simulink model "BaseEngineController_LS"  (Simulink 7.7)
settings: Solver=FixedStepDiscrete  StartTime=0.0  StopTime=10.0  RelTol=1e-3
PreLoadFcn:
  | try, eval([bdroot '_setup']); catch, eval('model_setup', ''); end
InitFcn:
  | try, eval([bdroot '_setup']); catch, eval('model_setup', ''); end
undefined symbols (not defined in the file): ECU555, High, motohawk_build_version, motohawk_trunc_name, motohawk_vardec_config_group, motohawk_vardec_path, True
libraries: MotoHawk_lib x1418, motohawk_control_primitives_lib x183, motohawk_engine_lib x32, simulink x21, motohawk_annotations_lib x9, AutoDoc_lib x8, simulink_extras x4, motohawk_ccp_examples_lib x1, motohawk_control_primitives_motoshare_lib x1
(part 19 of 27)

== system BaseEngineController_LS/Foreground/Control/ActuatorCharacterization/SequenceCutPattern/Hard Cycle Cut Pattern/Cycle4CutPatter ==
  Mux1 : Mux  Inputs=8
  motohawk_calibration10 : MotoHawk_lib/Calibration & Probing Blocks/motohawk_calibration  nam='HardCycle4Cyl4'  val=0  storage=Calibration  show_more=on  name_source=Use Parameter  data_type=int8  read_level=1  write_level=1  ovr_cals=on  view_as=Enumeration  enum_struct={'Enable', 'Cut'}  vector_style=Wide Row  use_help_units=on  help=''  units=''  use_header_enum=off  row_header_enum={}  col_header_enum={}  use_min_max=off  min_val=-inf  max_val=inf  use_precision=off  precision=''  gain=1  offset=0  exp=1  use_mototune_group=on  mototune_group=motohawk_vardec_path(gcb)
  motohawk_calibration11 : MotoHawk_lib/Calibration & Probing Blocks/motohawk_calibration  nam='HardCycle4Cyl1'  val=1  storage=Calibration  show_more=on  name_source=Use Parameter  data_type=int8  read_level=1  write_level=1  ovr_cals=on  view_as=Enumeration  enum_struct={'Enable', 'Cut'}  vector_style=Wide Row  use_help_units=on  help=''  units=''  use_header_enum=off  row_header_enum={}  col_header_enum={}  use_min_max=off  min_val=-inf  max_val=inf  use_precision=off  precision=''  gain=1  offset=0  exp=1  use_mototune_group=on  mototune_group=motohawk_vardec_path(gcb)
  motohawk_calibration12 : MotoHawk_lib/Calibration & Probing Blocks/motohawk_calibration  nam='HardCycle4Cyl5'  val=1  storage=Calibration  show_more=on  name_source=Use Parameter  data_type=int8  read_level=1  write_level=1  ovr_cals=on  view_as=Enumeration  enum_struct={'Enable', 'Cut'}  vector_style=Wide Row  use_help_units=on  help=''  units=''  use_header_enum=off  row_header_enum={}  col_header_enum={}  use_min_max=off  min_val=-inf  max_val=inf  use_precision=off  precision=''  gain=1  offset=0  exp=1  use_mototune_group=on  mototune_group=motohawk_vardec_path(gcb)
  motohawk_calibration13 : MotoHawk_lib/Calibration & Probing Blocks/motohawk_calibration  nam='HardCycle4Cyl6'  val=1  storage=Calibration  show_more=on  name_source=Use Parameter  data_type=int8  read_level=1  write_level=1  ovr_cals=on  view_as=Enumeration  enum_struct={'Enable', 'Cut'}  vector_style=Wide Row  use_help_units=on  help=''  units=''  use_header_enum=off  row_header_enum={}  col_header_enum={}  use_min_max=off  min_val=-inf  max_val=inf  use_precision=off  precision=''  gain=1  offset=0  exp=1  use_mototune_group=on  mototune_group=motohawk_vardec_path(gcb)
  motohawk_calibration14 : MotoHawk_lib/Calibration & Probing Blocks/motohawk_calibration  nam='HardCycle4Cyl7'  val=1  storage=Calibration  show_more=on  name_source=Use Parameter  data_type=int8  read_level=1  write_level=1  ovr_cals=on  view_as=Enumeration  enum_struct={'Enable', 'Cut'}  vector_style=Wide Row  use_help_units=on  help=''  units=''  use_header_enum=off  row_header_enum={}  col_header_enum={}  use_min_max=off  min_val=-inf  max_val=inf  use_precision=off  precision=''  gain=1  offset=0  exp=1  use_mototune_group=on  mototune_group=motohawk_vardec_path(gcb)
  motohawk_calibration15 : MotoHawk_lib/Calibration & Probing Blocks/motohawk_calibration  nam='HardCycle4Cyl8'  val=1  storage=Calibration  show_more=on  name_source=Use Parameter  data_type=int8  read_level=1  write_level=1  ovr_cals=on  view_as=Enumeration  enum_struct={'Enable', 'Cut'}  vector_style=Wide Row  use_help_units=on  help=''  units=''  use_header_enum=off  row_header_enum={}  col_header_enum={}  use_min_max=off  min_val=-inf  max_val=inf  use_precision=off  precision=''  gain=1  offset=0  exp=1  use_mototune_group=on  mototune_group=motohawk_vardec_path(gcb)
  motohawk_calibration8 : MotoHawk_lib/Calibration & Probing Blocks/motohawk_calibration  nam='HardCycle4Cyl2'  val=1  storage=Calibration  show_more=on  name_source=Use Parameter  data_type=int8  read_level=1  write_level=1  ovr_cals=on  view_as=Enumeration  enum_struct={'Enable', 'Cut'}  vector_style=Wide Row  use_help_units=on  help=''  units=''  use_header_enum=off  row_header_enum={}  col_header_enum={}  use_min_max=off  min_val=-inf  max_val=inf  use_precision=off  precision=''  gain=1  offset=0  exp=1  use_mototune_group=on  mototune_group=motohawk_vardec_path(gcb)
  motohawk_calibration9 : MotoHawk_lib/Calibration & Probing Blocks/motohawk_calibration  nam='HardCycle4Cyl3'  val=1  storage=Calibration  show_more=on  name_source=Use Parameter  data_type=int8  read_level=1  write_level=1  ovr_cals=on  view_as=Enumeration  enum_struct={'Enable', 'Cut'}  vector_style=Wide Row  use_help_units=on  help=''  units=''  use_header_enum=off  row_header_enum={}  col_header_enum={}  use_min_max=off  min_val=-inf  max_val=inf  use_precision=off  precision=''  gain=1  offset=0  exp=1  use_mototune_group=on  mototune_group=motohawk_vardec_path(gcb)
  Out : Outport
  wires:
  Mux1/1 -> Out/1
  motohawk_calibration15/1 -> Mux1/8
  motohawk_calibration14/1 -> Mux1/7
  motohawk_calibration13/1 -> Mux1/6
  motohawk_calibration12/1 -> Mux1/5
  motohawk_calibration10/1 -> Mux1/4
  motohawk_calibration9/1 -> Mux1/3
  motohawk_calibration8/1 -> Mux1/2
  motohawk_calibration11/1 -> Mux1/1

== system BaseEngineController_LS/Foreground/Control/ActuatorCharacterization/SequenceCutPattern/Medium Cycle Cut Pattern/Cycle1CutPatter ==
  Mux1 : Mux  Inputs=8
  motohawk_calibration10 : MotoHawk_lib/Calibration & Probing Blocks/motohawk_calibration  nam='MediumCycle1Cyl4'  val=0  storage=Calibration  show_more=on  name_source=Use Parameter  data_type=int8  read_level=1  write_level=1  ovr_cals=on  view_as=Enumeration  enum_struct={'Enable', 'Cut'}  vector_style=Wide Row  use_help_units=on  help=''  units=''  use_header_enum=off  row_header_enum={}  col_header_enum={}  use_min_max=off  min_val=-inf  max_val=inf  use_precision=off  precision=''  gain=1  offset=0  exp=1  use_mototune_group=on  mototune_group=motohawk_vardec_path(gcb)
  motohawk_calibration11 : MotoHawk_lib/Calibration & Probing Blocks/motohawk_calibration  nam='MediumCycle1Cyl1'  val=1  storage=Calibration  show_more=on  name_source=Use Parameter  data_type=int8  read_level=1  write_level=1  ovr_cals=on  view_as=Enumeration  enum_struct={'Enable', 'Cut'}  vector_style=Wide Row  use_help_units=on  help=''  units=''  use_header_enum=off  row_header_enum={}  col_header_enum={}  use_min_max=off  min_val=-inf  max_val=inf  use_precision=off  precision=''  gain=1  offset=0  exp=1  use_mototune_group=on  mototune_group=motohawk_vardec_path(gcb)
  motohawk_calibration12 : MotoHawk_lib/Calibration & Probing Blocks/motohawk_calibration  nam='MediumCycle1Cyl5'  val=1  storage=Calibration  show_more=on  name_source=Use Parameter  data_type=int8  read_level=1  write_level=1  ovr_cals=on  view_as=Enumeration  enum_struct={'Enable', 'Cut'}  vector_style=Wide Row  use_help_units=on  help=''  units=''  use_header_enum=off  row_header_enum={}  col_header_enum={}  use_min_max=off  min_val=-inf  max_val=inf  use_precision=off  precision=''  gain=1  offset=0  exp=1  use_mototune_group=on  mototune_group=motohawk_vardec_path(gcb)
  motohawk_calibration13 : MotoHawk_lib/Calibration & Probing Blocks/motohawk_calibration  nam='MediumCycle1Cyl6'  val=1  storage=Calibration  show_more=on  name_source=Use Parameter  data_type=int8  read_level=1  write_level=1  ovr_cals=on  view_as=Enumeration  enum_struct={'Enable', 'Cut'}  vector_style=Wide Row  use_help_units=on  help=''  units=''  use_header_enum=off  row_header_enum={}  col_header_enum={}  use_min_max=off  min_val=-inf  max_val=inf  use_precision=off  precision=''  gain=1  offset=0  exp=1  use_mototune_group=on  mototune_group=motohawk_vardec_path(gcb)
  motohawk_calibration14 : MotoHawk_lib/Calibration & Probing Blocks/motohawk_calibration  nam='MediumCycle1Cyl7'  val=1  storage=Calibration  show_more=on  name_source=Use Parameter  data_type=int8  read_level=1  write_level=1  ovr_cals=on  view_as=Enumeration  enum_struct={'Enable', 'Cut'}  vector_style=Wide Row  use_help_units=on  help=''  units=''  use_header_enum=off  row_header_enum={}  col_header_enum={}  use_min_max=off  min_val=-inf  max_val=inf  use_precision=off  precision=''  gain=1  offset=0  exp=1  use_mototune_group=on  mototune_group=motohawk_vardec_path(gcb)
  motohawk_calibration15 : MotoHawk_lib/Calibration & Probing Blocks/motohawk_calibration  nam='MediumCycle1Cyl8'  val=1  storage=Calibration  show_more=on  name_source=Use Parameter  data_type=int8  read_level=1  write_level=1  ovr_cals=on  view_as=Enumeration  enum_struct={'Enable', 'Cut'}  vector_style=Wide Row  use_help_units=on  help=''  units=''  use_header_enum=off  row_header_enum={}  col_header_enum={}  use_min_max=off  min_val=-inf  max_val=inf  use_precision=off  precision=''  gain=1  offset=0  exp=1  use_mototune_group=on  mototune_group=motohawk_vardec_path(gcb)
  motohawk_calibration8 : MotoHawk_lib/Calibration & Probing Blocks/motohawk_calibration  nam='MediumCycle1Cyl2'  val=1  storage=Calibration  show_more=on  name_source=Use Parameter  data_type=int8  read_level=1  write_level=1  ovr_cals=on  view_as=Enumeration  enum_struct={'Enable', 'Cut'}  vector_style=Wide Row  use_help_units=on  help=''  units=''  use_header_enum=off  row_header_enum={}  col_header_enum={}  use_min_max=off  min_val=-inf  max_val=inf  use_precision=off  precision=''  gain=1  offset=0  exp=1  use_mototune_group=on  mototune_group=motohawk_vardec_path(gcb)
  motohawk_calibration9 : MotoHawk_lib/Calibration & Probing Blocks/motohawk_calibration  nam='MediumCycle1Cyl3'  val=0  storage=Calibration  show_more=on  name_source=Use Parameter  data_type=int8  read_level=1  write_level=1  ovr_cals=on  view_as=Enumeration  enum_struct={'Enable', 'Cut'}  vector_style=Wide Row  use_help_units=on  help=''  units=''  use_header_enum=off  row_header_enum={}  col_header_enum={}  use_min_max=off  min_val=-inf  max_val=inf  use_precision=off  precision=''  gain=1  offset=0  exp=1  use_mototune_group=on  mototune_group=motohawk_vardec_path(gcb)
  Out : Outport
  wires:
  Mux1/1 -> Out/1
  motohawk_calibration15/1 -> Mux1/8
  motohawk_calibration14/1 -> Mux1/7
  motohawk_calibration13/1 -> Mux1/6
  motohawk_calibration12/1 -> Mux1/5
  motohawk_calibration10/1 -> Mux1/4
  motohawk_calibration9/1 -> Mux1/3
  motohawk_calibration8/1 -> Mux1/2
  motohawk_calibration11/1 -> Mux1/1

== system BaseEngineController_LS/Foreground/Control/ActuatorCharacterization/SequenceCutPattern/Medium Cycle Cut Pattern/Cycle2CutPatter ==
  Mux1 : Mux  Inputs=8
  motohawk_calibration10 : MotoHawk_lib/Calibration & Probing Blocks/motohawk_calibration  nam='MediumCycle2Cyl4'  val=1  storage=Calibration  show_more=on  name_source=Use Parameter  data_type=int8  read_level=1  write_level=1  ovr_cals=on  view_as=Enumeration  enum_struct={'Enable', 'Cut'}  vector_style=Wide Row  use_help_units=on  help=''  units=''  use_header_enum=off  row_header_enum={}  col_header_enum={}  use_min_max=off  min_val=-inf  max_val=inf  use_precision=off  precision=''  gain=1  offset=0  exp=1  use_mototune_group=on  mototune_group=motohawk_vardec_path(gcb)
  motohawk_calibration11 : MotoHawk_lib/Calibration & Probing Blocks/motohawk_calibration  nam='MediumCycle2Cyl1'  val=0  storage=Calibration  show_more=on  name_source=Use Parameter  data_type=int8  read_level=1  write_level=1  ovr_cals=on  view_as=Enumeration  enum_struct={'Enable', 'Cut'}  vector_style=Wide Row  use_help_units=on  help=''  units=''  use_header_enum=off  row_header_enum={}  col_header_enum={}  use_min_max=off  min_val=-inf  max_val=inf  use_precision=off  precision=''  gain=1  offset=0  exp=1  use_mototune_group=on  mototune_group=motohawk_vardec_path(gcb)
  motohawk_calibration12 : MotoHawk_lib/Calibration & Probing Blocks/motohawk_calibration  nam='MediumCycle2Cyl5'  val=1  storage=Calibration  show_more=on  name_source=Use Parameter  data_type=int8  read_level=1  write_level=1  ovr_cals=on  view_as=Enumeration  enum_struct={'Enable', 'Cut'}  vector_style=Wide Row  use_help_units=on  help=''  units=''  use_header_enum=off  row_header_enum={}  col_header_enum={}  use_min_max=off  min_val=-inf  max_val=inf  use_precision=off  precision=''  gain=1  offset=0  exp=1  use_mototune_group=on  mototune_group=motohawk_vardec_path(gcb)
  motohawk_calibration13 : MotoHawk_lib/Calibration & Probing Blocks/motohawk_calibration  nam='MediumCycle2Cyl6'  val=1  storage=Calibration  show_more=on  name_source=Use Parameter  data_type=int8  read_level=1  write_level=1  ovr_cals=on  view_as=Enumeration  enum_struct={'Enable', 'Cut'}  vector_style=Wide Row  use_help_units=on  help=''  units=''  use_header_enum=off  row_header_enum={}  col_header_enum={}  use_min_max=off  min_val=-inf  max_val=inf  use_precision=off  precision=''  gain=1  offset=0  exp=1  use_mototune_group=on  mototune_group=motohawk_vardec_path(gcb)
  motohawk_calibration14 : MotoHawk_lib/Calibration & Probing Blocks/motohawk_calibration  nam='MediumCycle2Cyl7'  val=1  storage=Calibration  show_more=on  name_source=Use Parameter  data_type=int8  read_level=1  write_level=1  ovr_cals=on  view_as=Enumeration  enum_struct={'Enable', 'Cut'}  vector_style=Wide Row  use_help_units=on  help=''  units=''  use_header_enum=off  row_header_enum={}  col_header_enum={}  use_min_max=off  min_val=-inf  max_val=inf  use_precision=off  precision=''  gain=1  offset=0  exp=1  use_mototune_group=on  mototune_group=motohawk_vardec_path(gcb)
  motohawk_calibration15 : MotoHawk_lib/Calibration & Probing Blocks/motohawk_calibration  nam='MediumCycle2Cyl8'  val=1  storage=Calibration  show_more=on  name_source=Use Parameter  data_type=int8  read_level=1  write_level=1  ovr_cals=on  view_as=Enumeration  enum_struct={'Enable', 'Cut'}  vector_style=Wide Row  use_help_units=on  help=''  units=''  use_header_enum=off  row_header_enum={}  col_header_enum={}  use_min_max=off  min_val=-inf  max_val=inf  use_precision=off  precision=''  gain=1  offset=0  exp=1  use_mototune_group=on  mototune_group=motohawk_vardec_path(gcb)
  motohawk_calibration8 : MotoHawk_lib/Calibration & Probing Blocks/motohawk_calibration  nam='MediumCycle2Cyl2'  val=0  storage=Calibration  show_more=on  name_source=Use Parameter  data_type=int8  read_level=1  write_level=1  ovr_cals=on  view_as=Enumeration  enum_struct={'Enable', 'Cut'}  vector_style=Wide Row  use_help_units=on  help=''  units=''  use_header_enum=off  row_header_enum={}  col_header_enum={}  use_min_max=off  min_val=-inf  max_val=inf  use_precision=off  precision=''  gain=1  offset=0  exp=1  use_mototune_group=on  mototune_group=motohawk_vardec_path(gcb)
  motohawk_calibration9 : MotoHawk_lib/Calibration & Probing Blocks/motohawk_calibration  nam='MediumCycle2Cyl3'  val=1  storage=Calibration  show_more=on  name_source=Use Parameter  data_type=int8  read_level=1  write_level=1  ovr_cals=on  view_as=Enumeration  enum_struct={'Enable', 'Cut'}  vector_style=Wide Row  use_help_units=on  help=''  units=''  use_header_enum=off  row_header_enum={}  col_header_enum={}  use_min_max=off  min_val=-inf  max_val=inf  use_precision=off  precision=''  gain=1  offset=0  exp=1  use_mototune_group=on  mototune_group=motohawk_vardec_path(gcb)
  Out : Outport
  wires:
  motohawk_calibration11/1 -> Mux1/1
  motohawk_calibration8/1 -> Mux1/2
  motohawk_calibration9/1 -> Mux1/3
  motohawk_calibration10/1 -> Mux1/4
  motohawk_calibration12/1 -> Mux1/5
  motohawk_calibration13/1 -> Mux1/6
  motohawk_calibration14/1 -> Mux1/7
  motohawk_calibration15/1 -> Mux1/8
  Mux1/1 -> Out/1

== system BaseEngineController_LS/Foreground/Control/ActuatorCharacterization/SequenceCutPattern/Medium Cycle Cut Pattern/Cycle3CutPatter ==
  Mux1 : Mux  Inputs=8
  motohawk_calibration10 : MotoHawk_lib/Calibration & Probing Blocks/motohawk_calibration  nam='MediumCycle3Cyl4'  val=0  storage=Calibration  show_more=on  name_source=Use Parameter  data_type=int8  read_level=1  write_level=1  ovr_cals=on  view_as=Enumeration  enum_struct={'Enable', 'Cut'}  vector_style=Wide Row  use_help_units=on  help=''  units=''  use_header_enum=off  row_header_enum={}  col_header_enum={}  use_min_max=off  min_val=-inf  max_val=inf  use_precision=off  precision=''  gain=1  offset=0  exp=1  use_mototune_group=on  mototune_group=motohawk_vardec_path(gcb)
  motohawk_calibration11 : MotoHawk_lib/Calibration & Probing Blocks/motohawk_calibration  nam='MediumCycle3Cyl1'  val=1  storage=Calibration  show_more=on  name_source=Use Parameter  data_type=int8  read_level=1  write_level=1  ovr_cals=on  view_as=Enumeration  enum_struct={'Enable', 'Cut'}  vector_style=Wide Row  use_help_units=on  help=''  units=''  use_header_enum=off  row_header_enum={}  col_header_enum={}  use_min_max=off  min_val=-inf  max_val=inf  use_precision=off  precision=''  gain=1  offset=0  exp=1  use_mototune_group=on  mototune_group=motohawk_vardec_path(gcb)
  motohawk_calibration12 : MotoHawk_lib/Calibration & Probing Blocks/motohawk_calibration  nam='MediumCycle3Cyl5'  val=1  storage=Calibration  show_more=on  name_source=Use Parameter  data_type=int8  read_level=1  write_level=1  ovr_cals=on  view_as=Enumeration  enum_struct={'Enable', 'Cut'}  vector_style=Wide Row  use_help_units=on  help=''  units=''  use_header_enum=off  row_header_enum={}  col_header_enum={}  use_min_max=off  min_val=-inf  max_val=inf  use_precision=off  precision=''  gain=1  offset=0  exp=1  use_mototune_group=on  mototune_group=motohawk_vardec_path(gcb)
  motohawk_calibration13 : MotoHawk_lib/Calibration & Probing Blocks/motohawk_calibration  nam='MediumCycle3Cyl6'  val=1  storage=Calibration  show_more=on  name_source=Use Parameter  data_type=int8  read_level=1  write_level=1  ovr_cals=on  view_as=Enumeration  enum_struct={'Enable', 'Cut'}  vector_style=Wide Row  use_help_units=on  help=''  units=''  use_header_enum=off  row_header_enum={}  col_header_enum={}  use_min_max=off  min_val=-inf  max_val=inf  use_precision=off  precision=''  gain=1  offset=0  exp=1  use_mototune_group=on  mototune_group=motohawk_vardec_path(gcb)
  motohawk_calibration14 : MotoHawk_lib/Calibration & Probing Blocks/motohawk_calibration  nam='MediumCycle3Cyl7'  val=1  storage=Calibration  show_more=on  name_source=Use Parameter  data_type=int8  read_level=1  write_level=1  ovr_cals=on  view_as=Enumeration  enum_struct={'Enable', 'Cut'}  vector_style=Wide Row  use_help_units=on  help=''  units=''  use_header_enum=off  row_header_enum={}  col_header_enum={}  use_min_max=off  min_val=-inf  max_val=inf  use_precision=off  precision=''  gain=1  offset=0  exp=1  use_mototune_group=on  mototune_group=motohawk_vardec_path(gcb)
  motohawk_calibration15 : MotoHawk_lib/Calibration & Probing Blocks/motohawk_calibration  nam='MediumCycle3Cyl8'  val=1  storage=Calibration  show_more=on  name_source=Use Parameter  data_type=int8  read_level=1  write_level=1  ovr_cals=on  view_as=Enumeration  enum_struct={'Enable', 'Cut'}  vector_style=Wide Row  use_help_units=on  help=''  units=''  use_header_enum=off  row_header_enum={}  col_header_enum={}  use_min_max=off  min_val=-inf  max_val=inf  use_precision=off  precision=''  gain=1  offset=0  exp=1  use_mototune_group=on  mototune_group=motohawk_vardec_path(gcb)
  motohawk_calibration8 : MotoHawk_lib/Calibration & Probing Blocks/motohawk_calibration  nam='MediumCycle3Cyl2'  val=0  storage=Calibration  show_more=on  name_source=Use Parameter  data_type=int8  read_level=1  write_level=1  ovr_cals=on  view_as=Enumeration  enum_struct={'Enable', 'Cut'}  vector_style=Wide Row  use_help_units=on  help=''  units=''  use_header_enum=off  row_header_enum={}  col_header_enum={}  use_min_max=off  min_val=-inf  max_val=inf  use_precision=off  precision=''  gain=1  offset=0  exp=1  use_mototune_group=on  mototune_group=motohawk_vardec_path(gcb)
  motohawk_calibration9 : MotoHawk_lib/Calibration & Probing Blocks/motohawk_calibration  nam='MediumCycle3Cyl3'  val=1  storage=Calibration  show_more=on  name_source=Use Parameter  data_type=int8  read_level=1  write_level=1  ovr_cals=on  view_as=Enumeration  enum_struct={'Enable', 'Cut'}  vector_style=Wide Row  use_help_units=on  help=''  units=''  use_header_enum=off  row_header_enum={}  col_header_enum={}  use_min_max=off  min_val=-inf  max_val=inf  use_precision=off  precision=''  gain=1  offset=0  exp=1  use_mototune_group=on  mototune_group=motohawk_vardec_path(gcb)
  Out : Outport
  wires:
  Mux1/1 -> Out/1
  motohawk_calibration15/1 -> Mux1/8
  motohawk_calibration14/1 -> Mux1/7
  motohawk_calibration13/1 -> Mux1/6
  motohawk_calibration12/1 -> Mux1/5
  motohawk_calibration10/1 -> Mux1/4
  motohawk_calibration9/1 -> Mux1/3
  motohawk_calibration8/1 -> Mux1/2
  motohawk_calibration11/1 -> Mux1/1

== system BaseEngineController_LS/Foreground/Control/ActuatorCharacterization/SequenceCutPattern/Medium Cycle Cut Pattern/Cycle4CutPatter ==
  Mux1 : Mux  Inputs=8
  motohawk_calibration10 : MotoHawk_lib/Calibration & Probing Blocks/motohawk_calibration  nam='MediumCycle4Cyl4'  val=0  storage=Calibration  show_more=on  name_source=Use Parameter  data_type=int8  read_level=1  write_level=1  ovr_cals=on  view_as=Enumeration  enum_struct={'Enable', 'Cut'}  vector_style=Wide Row  use_help_units=on  help=''  units=''  use_header_enum=off  row_header_enum={}  col_header_enum={}  use_min_max=off  min_val=-inf  max_val=inf  use_precision=off  precision=''  gain=1  offset=0  exp=1  use_mototune_group=on  mototune_group=motohawk_vardec_path(gcb)
  motohawk_calibration11 : MotoHawk_lib/Calibration & Probing Blocks/motohawk_calibration  nam='MediumCycle4Cyl1'  val=0  storage=Calibration  show_more=on  name_source=Use Parameter  data_type=int8  read_level=1  write_level=1  ovr_cals=on  view_as=Enumeration  enum_struct={'Enable', 'Cut'}  vector_style=Wide Row  use_help_units=on  help=''  units=''  use_header_enum=off  row_header_enum={}  col_header_enum={}  use_min_max=off  min_val=-inf  max_val=inf  use_precision=off  precision=''  gain=1  offset=0  exp=1  use_mototune_group=on  mototune_group=motohawk_vardec_path(gcb)
  motohawk_calibration12 : MotoHawk_lib/Calibration & Probing Blocks/motohawk_calibration  nam='MediumCycle4Cyl5'  val=1  storage=Calibration  show_more=on  name_source=Use Parameter  data_type=int8  read_level=1  write_level=1  ovr_cals=on  view_as=Enumeration  enum_struct={'Enable', 'Cut'}  vector_style=Wide Row  use_help_units=on  help=''  units=''  use_header_enum=off  row_header_enum={}  col_header_enum={}  use_min_max=off  min_val=-inf  max_val=inf  use_precision=off  precision=''  gain=1  offset=0  exp=1  use_mototune_group=on  mototune_group=motohawk_vardec_path(gcb)
  motohawk_calibration13 : MotoHawk_lib/Calibration & Probing Blocks/motohawk_calibration  nam='MediumCycle4Cyl6'  val=1  storage=Calibration  show_more=on  name_source=Use Parameter  data_type=int8  read_level=1  write_level=1  ovr_cals=on  view_as=Enumeration  enum_struct={'Enable', 'Cut'}  vector_style=Wide Row  use_help_units=on  help=''  units=''  use_header_enum=off  row_header_enum={}  col_header_enum={}  use_min_max=off  min_val=-inf  max_val=inf  use_precision=off  precision=''  gain=1  offset=0  exp=1  use_mototune_group=on  mototune_group=motohawk_vardec_path(gcb)
  motohawk_calibration14 : MotoHawk_lib/Calibration & Probing Blocks/motohawk_calibration  nam='MediumCycle4Cyl7'  val=1  storage=Calibration  show_more=on  name_source=Use Parameter  data_type=int8  read_level=1  write_level=1  ovr_cals=on  view_as=Enumeration  enum_struct={'Enable', 'Cut'}  vector_style=Wide Row  use_help_units=on  help=''  units=''  use_header_enum=off  row_header_enum={}  col_header_enum={}  use_min_max=off  min_val=-inf  max_val=inf  use_precision=off  precision=''  gain=1  offset=0  exp=1  use_mototune_group=on  mototune_group=motohawk_vardec_path(gcb)
  motohawk_calibration15 : MotoHawk_lib/Calibration & Probing Blocks/motohawk_calibration  nam='MediumCycle4Cyl8'  val=1  storage=Calibration  show_more=on  name_source=Use Parameter  data_type=int8  read_level=1  write_level=1  ovr_cals=on  view_as=Enumeration  enum_struct={'Enable', 'Cut'}  vector_style=Wide Row  use_help_units=on  help=''  units=''  use_header_enum=off  row_header_enum={}  col_header_enum={}  use_min_max=off  min_val=-inf  max_val=inf  use_precision=off  precision=''  gain=1  offset=0  exp=1  use_mototune_group=on  mototune_group=motohawk_vardec_path(gcb)
  motohawk_calibration8 : MotoHawk_lib/Calibration & Probing Blocks/motohawk_calibration  nam='MediumCycle4Cyl2'  val=1  storage=Calibration  show_more=on  name_source=Use Parameter  data_type=int8  read_level=1  write_level=1  ovr_cals=on  view_as=Enumeration  enum_struct={'Enable', 'Cut'}  vector_style=Wide Row  use_help_units=on  help=''  units=''  use_header_enum=off  row_header_enum={}  col_header_enum={}  use_min_max=off  min_val=-inf  max_val=inf  use_precision=off  precision=''  gain=1  offset=0  exp=1  use_mototune_group=on  mototune_group=motohawk_vardec_path(gcb)
  motohawk_calibration9 : MotoHawk_lib/Calibration & Probing Blocks/motohawk_calibration  nam='MediumCycle4Cyl3'  val=1  storage=Calibration  show_more=on  name_source=Use Parameter  data_type=int8  read_level=1  write_level=1  ovr_cals=on  view_as=Enumeration  enum_struct={'Enable', 'Cut'}  vector_style=Wide Row  use_help_units=on  help=''  units=''  use_header_enum=off  row_header_enum={}  col_header_enum={}  use_min_max=off  min_val=-inf  max_val=inf  use_precision=off  precision=''  gain=1  offset=0  exp=1  use_mototune_group=on  mototune_group=motohawk_vardec_path(gcb)
  Out : Outport
  wires:
  motohawk_calibration11/1 -> Mux1/1
  motohawk_calibration8/1 -> Mux1/2
  motohawk_calibration9/1 -> Mux1/3
  motohawk_calibration10/1 -> Mux1/4
  motohawk_calibration12/1 -> Mux1/5
  motohawk_calibration13/1 -> Mux1/6
  motohawk_calibration14/1 -> Mux1/7
  motohawk_calibration15/1 -> Mux1/8
  Mux1/1 -> Out/1

== system BaseEngineController_LS/Foreground/Control/ActuatorCharacterization/SequenceCutPattern/SequenceCutMachine/SequencyCutMachine ==
  note: Counter Increment
  note: CounterReset
  CutArray : Inport
  CurrentCount : Inport  Port=2
  CurrentCycle : Inport  Port=3
  function : TriggerPort  TriggerType=function-call
  Constant : Constant  OutDataTypeStr=uint8  SampleTime=-1
  Constant1 : Constant  Value=4  OutDataTypeStr=uint8  SampleTime=-1
  Constant10 : Constant  OutDataTypeStr=uint8  SampleTime=-1
  Constant11 : Constant  Value=5  OutDataTypeStr=uint8  SampleTime=-1
  Constant2 : Constant  Value=5  OutDataTypeStr=uint8  SampleTime=-1
  Constant3 : Constant  OutDataTypeStr=uint8  SampleTime=-1
  Relational Operator : RelationalOperator  Operator=<=
  Relational Operator1 : RelationalOperator  Operator===  OutDataTypeStr=uint(8)
  Relational Operator2 : RelationalOperator  Operator=<=
  Sum1 : Sum  SaturateOnIntegerOverflow=on
  Sum2 : Sum  SaturateOnIntegerOverflow=on
  Switch : Switch  Threshold=1  SaturateOnIntegerOverflow=on
  Switch1 : Switch  Threshold=1  SaturateOnIntegerOverflow=on
  CylsToCut : Outport
  CycleCounter : Outport  Port=2  InitialOutput=1
  CycleNumber : Outport  Port=3  InitialOutput=1
  wires:
  CutArray/1 -> CylsToCut/1
  CurrentCount/1 -> Sum1/1
  Constant/1 -> Sum1/2
  Relational Operator/1 -> Switch/2
  Sum1/1 -> Switch/3, Relational Operator/2
  Constant10/1 -> Switch/1
  Constant11/1 -> Relational Operator/1
  Switch/1 -> CycleCounter/1, Relational Operator1/1
  CurrentCycle/1 -> Sum2/2
  Relational Operator1/1 -> Sum2/1
  Constant1/1 -> Relational Operator1/2
  Switch1/1 -> CycleNumber/1
  Sum2/1 -> Switch1/3, Relational Operator2/2
  Relational Operator2/1 -> Switch1/2
  Constant2/1 -> Relational Operator2/1
  Constant3/1 -> Switch1/1

== system BaseEngineController_LS/Foreground/Control/ActuatorCharacterization/SequenceCutPattern/Soft Cycle Cut Pattern/Cycle1CutPatter ==
  Mux1 : Mux  Inputs=8
  motohawk_calibration10 : MotoHawk_lib/Calibration & Probing Blocks/motohawk_calibration  nam='SoftCycle1Cyl4'  val=0  storage=Calibration  show_more=on  name_source=Use Parameter  data_type=int8  read_level=1  write_level=1  ovr_cals=on  view_as=Enumeration  enum_struct={'Enable', 'Cut'}  vector_style=Wide Row  use_help_units=on  help=''  units=''  use_header_enum=off  row_header_enum={}  col_header_enum={}  use_min_max=off  min_val=-inf  max_val=inf  use_precision=off  precision=''  gain=1  offset=0  exp=1  use_mototune_group=on  mototune_group=motohawk_vardec_path(gcb)
  motohawk_calibration11 : MotoHawk_lib/Calibration & Probing Blocks/motohawk_calibration  nam='SoftCycle1Cyl1'  val=1  storage=Calibration  show_more=on  name_source=Use Parameter  data_type=int8  read_level=1  write_level=1  ovr_cals=on  view_as=Enumeration  enum_struct={'Enable', 'Cut'}  vector_style=Wide Row  use_help_units=on  help=''  units=''  use_header_enum=off  row_header_enum={}  col_header_enum={}  use_min_max=off  min_val=-inf  max_val=inf  use_precision=off  precision=''  gain=1  offset=0  exp=1  use_mototune_group=on  mototune_group=motohawk_vardec_path(gcb)
  motohawk_calibration12 : MotoHawk_lib/Calibration & Probing Blocks/motohawk_calibration  nam='SoftCycle1Cyl5'  val=1  storage=Calibration  show_more=on  name_source=Use Parameter  data_type=int8  read_level=1  write_level=1  ovr_cals=on  view_as=Enumeration  enum_struct={'Enable', 'Cut'}  vector_style=Wide Row  use_help_units=on  help=''  units=''  use_header_enum=off  row_header_enum={}  col_header_enum={}  use_min_max=off  min_val=-inf  max_val=inf  use_precision=off  precision=''  gain=1  offset=0  exp=1  use_mototune_group=on  mototune_group=motohawk_vardec_path(gcb)
  motohawk_calibration13 : MotoHawk_lib/Calibration & Probing Blocks/motohawk_calibration  nam='SoftCycle1Cyl6'  val=1  storage=Calibration  show_more=on  name_source=Use Parameter  data_type=int8  read_level=1  write_level=1  ovr_cals=on  view_as=Enumeration  enum_struct={'Enable', 'Cut'}  vector_style=Wide Row  use_help_units=on  help=''  units=''  use_header_enum=off  row_header_enum={}  col_header_enum={}  use_min_max=off  min_val=-inf  max_val=inf  use_precision=off  precision=''  gain=1  offset=0  exp=1  use_mototune_group=on  mototune_group=motohawk_vardec_path(gcb)
  motohawk_calibration14 : MotoHawk_lib/Calibration & Probing Blocks/motohawk_calibration  nam='SoftCycle1Cyl7'  val=1  storage=Calibration  show_more=on  name_source=Use Parameter  data_type=int8  read_level=1  write_level=1  ovr_cals=on  view_as=Enumeration  enum_struct={'Enable', 'Cut'}  vector_style=Wide Row  use_help_units=on  help=''  units=''  use_header_enum=off  row_header_enum={}  col_header_enum={}  use_min_max=off  min_val=-inf  max_val=inf  use_precision=off  precision=''  gain=1  offset=0  exp=1  use_mototune_group=on  mototune_group=motohawk_vardec_path(gcb)
  motohawk_calibration15 : MotoHawk_lib/Calibration & Probing Blocks/motohawk_calibration  nam='SoftCycle1Cyl8'  val=1  storage=Calibration  show_more=on  name_source=Use Parameter  data_type=int8  read_level=1  write_level=1  ovr_cals=on  view_as=Enumeration  enum_struct={'Enable', 'Cut'}  vector_style=Wide Row  use_help_units=on  help=''  units=''  use_header_enum=off  row_header_enum={}  col_header_enum={}  use_min_max=off  min_val=-inf  max_val=inf  use_precision=off  precision=''  gain=1  offset=0  exp=1  use_mototune_group=on  mototune_group=motohawk_vardec_path(gcb)
  motohawk_calibration8 : MotoHawk_lib/Calibration & Probing Blocks/motohawk_calibration  nam='SoftCycle1Cyl2'  val=0  storage=Calibration  show_more=on  name_source=Use Parameter  data_type=int8  read_level=1  write_level=1  ovr_cals=on  view_as=Enumeration  enum_struct={'Enable', 'Cut'}  vector_style=Wide Row  use_help_units=on  help=''  units=''  use_header_enum=off  row_header_enum={}  col_header_enum={}  use_min_max=off  min_val=-inf  max_val=inf  use_precision=off  precision=''  gain=1  offset=0  exp=1  use_mototune_group=on  mototune_group=motohawk_vardec_path(gcb)
  motohawk_calibration9 : MotoHawk_lib/Calibration & Probing Blocks/motohawk_calibration  nam='SoftCycle1Cyl3'  val=0  storage=Calibration  show_more=on  name_source=Use Parameter  data_type=int8  read_level=1  write_level=1  ovr_cals=on  view_as=Enumeration  enum_struct={'Enable', 'Cut'}  vector_style=Wide Row  use_help_units=on  help=''  units=''  use_header_enum=off  row_header_enum={}  col_header_enum={}  use_min_max=off  min_val=-inf  max_val=inf  use_precision=off  precision=''  gain=1  offset=0  exp=1  use_mototune_group=on  mototune_group=motohawk_vardec_path(gcb)
  Out : Outport
  wires:
  motohawk_calibration11/1 -> Mux1/1
  motohawk_calibration8/1 -> Mux1/2
  motohawk_calibration9/1 -> Mux1/3
  motohawk_calibration10/1 -> Mux1/4
  motohawk_calibration12/1 -> Mux1/5
  motohawk_calibration13/1 -> Mux1/6
  motohawk_calibration14/1 -> Mux1/7
  motohawk_calibration15/1 -> Mux1/8
  Mux1/1 -> Out/1

== system BaseEngineController_LS/Foreground/Control/ActuatorCharacterization/SequenceCutPattern/Soft Cycle Cut Pattern/Cycle2CutPatter ==
  Mux1 : Mux  Inputs=8
  motohawk_calibration10 : MotoHawk_lib/Calibration & Probing Blocks/motohawk_calibration  nam='SoftCycle2Cyl4'  val=0  storage=Calibration  show_more=on  name_source=Use Parameter  data_type=int8  read_level=1  write_level=1  ovr_cals=on  view_as=Enumeration  enum_struct={'Enable', 'Cut'}  vector_style=Wide Row  use_help_units=on  help=''  units=''  use_header_enum=off  row_header_enum={}  col_header_enum={}  use_min_max=off  min_val=-inf  max_val=inf  use_precision=off  precision=''  gain=1  offset=0  exp=1  use_mototune_group=on  mototune_group=motohawk_vardec_path(gcb)
  motohawk_calibration11 : MotoHawk_lib/Calibration & Probing Blocks/motohawk_calibration  nam='SoftCycle2Cyl1'  val=0  storage=Calibration  show_more=on  name_source=Use Parameter  data_type=int8  read_level=1  write_level=1  ovr_cals=on  view_as=Enumeration  enum_struct={'Enable', 'Cut'}  vector_style=Wide Row  use_help_units=on  help=''  units=''  use_header_enum=off  row_header_enum={}  col_header_enum={}  use_min_max=off  min_val=-inf  max_val=inf  use_precision=off  precision=''  gain=1  offset=0  exp=1  use_mototune_group=on  mototune_group=motohawk_vardec_path(gcb)
  motohawk_calibration12 : MotoHawk_lib/Calibration & Probing Blocks/motohawk_calibration  nam='SoftCycle2Cyl5'  val=1  storage=Calibration  show_more=on  name_source=Use Parameter  data_type=int8  read_level=1  write_level=1  ovr_cals=on  view_as=Enumeration  enum_struct={'Enable', 'Cut'}  vector_style=Wide Row  use_help_units=on  help=''  units=''  use_header_enum=off  row_header_enum={}  col_header_enum={}  use_min_max=off  min_val=-inf  max_val=inf  use_precision=off  precision=''  gain=1  offset=0  exp=1  use_mototune_group=on  mototune_group=motohawk_vardec_path(gcb)
  motohawk_calibration13 : MotoHawk_lib/Calibration & Probing Blocks/motohawk_calibration  nam='SoftCycle2Cyl6'  val=1  storage=Calibration  show_more=on  name_source=Use Parameter  data_type=int8  read_level=1  write_level=1  ovr_cals=on  view_as=Enumeration  enum_struct={'Enable', 'Cut'}  vector_style=Wide Row  use_help_units=on  help=''  units=''  use_header_enum=off  row_header_enum={}  col_header_enum={}  use_min_max=off  min_val=-inf  max_val=inf  use_precision=off  precision=''  gain=1  offset=0  exp=1  use_mototune_group=on  mototune_group=motohawk_vardec_path(gcb)
  motohawk_calibration14 : MotoHawk_lib/Calibration & Probing Blocks/motohawk_calibration  nam='SoftCycle2Cyl7'  val=1  storage=Calibration  show_more=on  name_source=Use Parameter  data_type=int8  read_level=1  write_level=1  ovr_cals=on  view_as=Enumeration  enum_struct={'Enable', 'Cut'}  vector_style=Wide Row  use_help_units=on  help=''  units=''  use_header_enum=off  row_header_enum={}  col_header_enum={}  use_min_max=off  min_val=-inf  max_val=inf  use_precision=off  precision=''  gain=1  offset=0  exp=1  use_mototune_group=on  mototune_group=motohawk_vardec_path(gcb)
  motohawk_calibration15 : MotoHawk_lib/Calibration & Probing Blocks/motohawk_calibration  nam='SoftCycle2Cyl8'  val=1  storage=Calibration  show_more=on  name_source=Use Parameter  data_type=int8  read_level=1  write_level=1  ovr_cals=on  view_as=Enumeration  enum_struct={'Enable', 'Cut'}  vector_style=Wide Row  use_help_units=on  help=''  units=''  use_header_enum=off  row_header_enum={}  col_header_enum={}  use_min_max=off  min_val=-inf  max_val=inf  use_precision=off  precision=''  gain=1  offset=0  exp=1  use_mototune_group=on  mototune_group=motohawk_vardec_path(gcb)
  motohawk_calibration8 : MotoHawk_lib/Calibration & Probing Blocks/motohawk_calibration  nam='SoftCycle2Cyl2'  val=1  storage=Calibration  show_more=on  name_source=Use Parameter  data_type=int8  read_level=1  write_level=1  ovr_cals=on  view_as=Enumeration  enum_struct={'Enable', 'Cut'}  vector_style=Wide Row  use_help_units=on  help=''  units=''  use_header_enum=off  row_header_enum={}  col_header_enum={}  use_min_max=off  min_val=-inf  max_val=inf  use_precision=off  precision=''  gain=1  offset=0  exp=1  use_mototune_group=on  mototune_group=motohawk_vardec_path(gcb)
  motohawk_calibration9 : MotoHawk_lib/Calibration & Probing Blocks/motohawk_calibration  nam='SoftCycle2Cyl3'  val=0  storage=Calibration  show_more=on  name_source=Use Parameter  data_type=int8  read_level=1  write_level=1  ovr_cals=on  view_as=Enumeration  enum_struct={'Enable', 'Cut'}  vector_style=Wide Row  use_help_units=on  help=''  units=''  use_header_enum=off  row_header_enum={}  col_header_enum={}  use_min_max=off  min_val=-inf  max_val=inf  use_precision=off  precision=''  gain=1  offset=0  exp=1  use_mototune_group=on  mototune_group=motohawk_vardec_path(gcb)
  Out : Outport
  wires:
  Mux1/1 -> Out/1
  motohawk_calibration15/1 -> Mux1/8
  motohawk_calibration14/1 -> Mux1/7
  motohawk_calibration13/1 -> Mux1/6
  motohawk_calibration12/1 -> Mux1/5
  motohawk_calibration10/1 -> Mux1/4
  motohawk_calibration9/1 -> Mux1/3
  motohawk_calibration8/1 -> Mux1/2
  motohawk_calibration11/1 -> Mux1/1

== system BaseEngineController_LS/Foreground/Control/ActuatorCharacterization/SequenceCutPattern/Soft Cycle Cut Pattern/Cycle3CutPatter ==
  Mux1 : Mux  Inputs=8
  motohawk_calibration10 : MotoHawk_lib/Calibration & Probing Blocks/motohawk_calibration  nam='SoftCycle3Cyl4'  val=0  storage=Calibration  show_more=on  name_source=Use Parameter  data_type=int8  read_level=1  write_level=1  ovr_cals=on  view_as=Enumeration  enum_struct={'Enable', 'Cut'}  vector_style=Wide Row  use_help_units=on  help=''  units=''  use_header_enum=off  row_header_enum={}  col_header_enum={}  use_min_max=off  min_val=-inf  max_val=inf  use_precision=off  precision=''  gain=1  offset=0  exp=1  use_mototune_group=on  mototune_group=motohawk_vardec_path(gcb)
  motohawk_calibration11 : MotoHawk_lib/Calibration & Probing Blocks/motohawk_calibration  nam='SoftCycle3Cyl1'  val=0  storage=Calibration  show_more=on  name_source=Use Parameter  data_type=int8  read_level=1  write_level=1  ovr_cals=on  view_as=Enumeration  enum_struct={'Enable', 'Cut'}  vector_style=Wide Row  use_help_units=on  help=''  units=''  use_header_enum=off  row_header_enum={}  col_header_enum={}  use_min_max=off  min_val=-inf  max_val=inf  use_precision=off  precision=''  gain=1  offset=0  exp=1  use_mototune_group=on  mototune_group=motohawk_vardec_path(gcb)
  motohawk_calibration12 : MotoHawk_lib/Calibration & Probing Blocks/motohawk_calibration  nam='SoftCycle3Cyl5'  val=1  storage=Calibration  show_more=on  name_source=Use Parameter  data_type=int8  read_level=1  write_level=1  ovr_cals=on  view_as=Enumeration  enum_struct={'Enable', 'Cut'}  vector_style=Wide Row  use_help_units=on  help=''  units=''  use_header_enum=off  row_header_enum={}  col_header_enum={}  use_min_max=off  min_val=-inf  max_val=inf  use_precision=off  precision=''  gain=1  offset=0  exp=1  use_mototune_group=on  mototune_group=motohawk_vardec_path(gcb)
  motohawk_calibration13 : MotoHawk_lib/Calibration & Probing Blocks/motohawk_calibration  nam='SoftCycle3Cyl6'  val=1  storage=Calibration  show_more=on  name_source=Use Parameter  data_type=int8  read_level=1  write_level=1  ovr_cals=on  view_as=Enumeration  enum_struct={'Enable', 'Cut'}  vector_style=Wide Row  use_help_units=on  help=''  units=''  use_header_enum=off  row_header_enum={}  col_header_enum={}  use_min_max=off  min_val=-inf  max_val=inf  use_precision=off  precision=''  gain=1  offset=0  exp=1  use_mototune_group=on  mototune_group=motohawk_vardec_path(gcb)
  motohawk_calibration14 : MotoHawk_lib/Calibration & Probing Blocks/motohawk_calibration  nam='SoftCycle3Cyl7'  val=1  storage=Calibration  show_more=on  name_source=Use Parameter  data_type=int8  read_level=1  write_level=1  ovr_cals=on  view_as=Enumeration  enum_struct={'Enable', 'Cut'}  vector_style=Wide Row  use_help_units=on  help=''  units=''  use_header_enum=off  row_header_enum={}  col_header_enum={}  use_min_max=off  min_val=-inf  max_val=inf  use_precision=off  precision=''  gain=1  offset=0  exp=1  use_mototune_group=on  mototune_group=motohawk_vardec_path(gcb)
  motohawk_calibration15 : MotoHawk_lib/Calibration & Probing Blocks/motohawk_calibration  nam='SoftCycle3Cyl8'  val=0  storage=Calibration  show_more=on  name_source=Use Parameter  data_type=int8  read_level=1  write_level=1  ovr_cals=on  view_as=Enumeration  enum_struct={'Enable', 'Cut'}  vector_style=Wide Row  use_help_units=on  help=''  units=''  use_header_enum=off  row_header_enum={}  col_header_enum={}  use_min_max=off  min_val=-inf  max_val=inf  use_precision=off  precision=''  gain=1  offset=0  exp=1  use_mototune_group=on  mototune_group=motohawk_vardec_path(gcb)
  motohawk_calibration8 : MotoHawk_lib/Calibration & Probing Blocks/motohawk_calibration  nam='SoftCycle3Cyl2'  val=0  storage=Calibration  show_more=on  name_source=Use Parameter  data_type=int8  read_level=1  write_level=1  ovr_cals=on  view_as=Enumeration  enum_struct={'Enable', 'Cut'}  vector_style=Wide Row  use_help_units=on  help=''  units=''  use_header_enum=off  row_header_enum={}  col_header_enum={}  use_min_max=off  min_val=-inf  max_val=inf  use_precision=off  precision=''  gain=1  offset=0  exp=1  use_mototune_group=on  mototune_group=motohawk_vardec_path(gcb)
  motohawk_calibration9 : MotoHawk_lib/Calibration & Probing Blocks/motohawk_calibration  nam='SoftCycle3Cyl3'  val=1  storage=Calibration  show_more=on  name_source=Use Parameter  data_type=int8  read_level=1  write_level=1  ovr_cals=on  view_as=Enumeration  enum_struct={'Enable', 'Cut'}  vector_style=Wide Row  use_help_units=on  help=''  units=''  use_header_enum=off  row_header_enum={}  col_header_enum={}  use_min_max=off  min_val=-inf  max_val=inf  use_precision=off  precision=''  gain=1  offset=0  exp=1  use_mototune_group=on  mototune_group=motohawk_vardec_path(gcb)
  Out : Outport
  wires:
  motohawk_calibration11/1 -> Mux1/1
  motohawk_calibration8/1 -> Mux1/2
  motohawk_calibration9/1 -> Mux1/3
  motohawk_calibration10/1 -> Mux1/4
  motohawk_calibration12/1 -> Mux1/5
  motohawk_calibration13/1 -> Mux1/6
  motohawk_calibration14/1 -> Mux1/7
  motohawk_calibration15/1 -> Mux1/8
  Mux1/1 -> Out/1

== system BaseEngineController_LS/Foreground/Control/ActuatorCharacterization/SequenceCutPattern/Soft Cycle Cut Pattern/Cycle4CutPatter ==
  Mux1 : Mux  Inputs=8
  motohawk_calibration10 : MotoHawk_lib/Calibration & Probing Blocks/motohawk_calibration  nam='SoftCycle4Cyl4'  val=1  storage=Calibration  show_more=on  name_source=Use Parameter  data_type=int8  read_level=1  write_level=1  ovr_cals=on  view_as=Enumeration  enum_struct={'Enable', 'Cut'}  vector_style=Wide Row  use_help_units=on  help=''  units=''  use_header_enum=off  row_header_enum={}  col_header_enum={}  use_min_max=off  min_val=-inf  max_val=inf  use_precision=off  precision=''  gain=1  offset=0  exp=1  use_mototune_group=on  mototune_group=motohawk_vardec_path(gcb)
  motohawk_calibration11 : MotoHawk_lib/Calibration & Probing Blocks/motohawk_calibration  nam='SoftCycle4Cyl1'  val=0  storage=Calibration  show_more=on  name_source=Use Parameter  data_type=int8  read_level=1  write_level=1  ovr_cals=on  view_as=Enumeration  enum_struct={'Enable', 'Cut'}  vector_style=Wide Row  use_help_units=on  help=''  units=''  use_header_enum=off  row_header_enum={}  col_header_enum={}  use_min_max=off  min_val=-inf  max_val=inf  use_precision=off  precision=''  gain=1  offset=0  exp=1  use_mototune_group=on  mototune_group=motohawk_vardec_path(gcb)
  motohawk_calibration12 : MotoHawk_lib/Calibration & Probing Blocks/motohawk_calibration  nam='SoftCycle4Cyl5'  val=1  storage=Calibration  show_more=on  name_source=Use Parameter  data_type=int8  read_level=1  write_level=1  ovr_cals=on  view_as=Enumeration  enum_struct={'Enable', 'Cut'}  vector_style=Wide Row  use_help_units=on  help=''  units=''  use_header_enum=off  row_header_enum={}  col_header_enum={}  use_min_max=off  min_val=-inf  max_val=inf  use_precision=off  precision=''  gain=1  offset=0  exp=1  use_mototune_group=on  mototune_group=motohawk_vardec_path(gcb)
  motohawk_calibration13 : MotoHawk_lib/Calibration & Probing Blocks/motohawk_calibration  nam='SoftCycle4Cyl6'  val=1  storage=Calibration  show_more=on  name_source=Use Parameter  data_type=int8  read_level=1  write_level=1  ovr_cals=on  view_as=Enumeration  enum_struct={'Enable', 'Cut'}  vector_style=Wide Row  use_help_units=on  help=''  units=''  use_header_enum=off  row_header_enum={}  col_header_enum={}  use_min_max=off  min_val=-inf  max_val=inf  use_precision=off  precision=''  gain=1  offset=0  exp=1  use_mototune_group=on  mototune_group=motohawk_vardec_path(gcb)
  motohawk_calibration14 : MotoHawk_lib/Calibration & Probing Blocks/motohawk_calibration  nam='SoftCycle4Cyl7'  val=1  storage=Calibration  show_more=on  name_source=Use Parameter  data_type=int8  read_level=1  write_level=1  ovr_cals=on  view_as=Enumeration  enum_struct={'Enable', 'Cut'}  vector_style=Wide Row  use_help_units=on  help=''  units=''  use_header_enum=off  row_header_enum={}  col_header_enum={}  use_min_max=off  min_val=-inf  max_val=inf  use_precision=off  precision=''  gain=1  offset=0  exp=1  use_mototune_group=on  mototune_group=motohawk_vardec_path(gcb)
  motohawk_calibration15 : MotoHawk_lib/Calibration & Probing Blocks/motohawk_calibration  nam='SoftCycle4Cyl8'  val=1  storage=Calibration  show_more=on  name_source=Use Parameter  data_type=int8  read_level=1  write_level=1  ovr_cals=on  view_as=Enumeration  enum_struct={'Enable', 'Cut'}  vector_style=Wide Row  use_help_units=on  help=''  units=''  use_header_enum=off  row_header_enum={}  col_header_enum={}  use_min_max=off  min_val=-inf  max_val=inf  use_precision=off  precision=''  gain=1  offset=0  exp=1  use_mototune_group=on  mototune_group=motohawk_vardec_path(gcb)
  motohawk_calibration8 : MotoHawk_lib/Calibration & Probing Blocks/motohawk_calibration  nam='SoftCycle4Cyl2'  val=0  storage=Calibration  show_more=on  name_source=Use Parameter  data_type=int8  read_level=1  write_level=1  ovr_cals=on  view_as=Enumeration  enum_struct={'Enable', 'Cut'}  vector_style=Wide Row  use_help_units=on  help=''  units=''  use_header_enum=off  row_header_enum={}  col_header_enum={}  use_min_max=off  min_val=-inf  max_val=inf  use_precision=off  precision=''  gain=1  offset=0  exp=1  use_mototune_group=on  mototune_group=motohawk_vardec_path(gcb)
  motohawk_calibration9 : MotoHawk_lib/Calibration & Probing Blocks/motohawk_calibration  nam='SoftCycle4Cyl3'  val=0  storage=Calibration  show_more=on  name_source=Use Parameter  data_type=int8  read_level=1  write_level=1  ovr_cals=on  view_as=Enumeration  enum_struct={'Enable', 'Cut'}  vector_style=Wide Row  use_help_units=on  help=''  units=''  use_header_enum=off  row_header_enum={}  col_header_enum={}  use_min_max=off  min_val=-inf  max_val=inf  use_precision=off  precision=''  gain=1  offset=0  exp=1  use_mototune_group=on  mototune_group=motohawk_vardec_path(gcb)
  Out : Outport
  wires:
  Mux1/1 -> Out/1
  motohawk_calibration15/1 -> Mux1/8
  motohawk_calibration14/1 -> Mux1/7
  motohawk_calibration13/1 -> Mux1/6
  motohawk_calibration12/1 -> Mux1/5
  motohawk_calibration10/1 -> Mux1/4
  motohawk_calibration9/1 -> Mux1/3
  motohawk_calibration8/1 -> Mux1/2
  motohawk_calibration11/1 -> Mux1/1

== system BaseEngineController_LS/Foreground/Control/Controller/Run/AC Control/AC Comp High Pressure ==
  HiThresh : Inport
  LowThresh : Inport  Port=2
  Signal : Inport  Port=3
  Hysteresis : Subsystem
  LT : RelationalOperator  ZeroCross=off  InputSameDT=on
  LT1 : RelationalOperator  Operator=<=  ZeroCross=off  InputSameDT=on
  Threshold : Outport
  wires:
  LT/1 -> Hysteresis/1(Hi)  "AboveHiTarget"
  LT1/1 -> Hysteresis/2(Lo)  "BelowLoTarget"
  Signal/1 -> LT/1, LT1/1
  Hysteresis/1("Out (Lo=0, Hi=1)") -> Threshold/1
  HiThresh/1 -> LT/2
  LowThresh/1 -> LT1/2
